simulink model "path_follower_req01"  (R2024a)
settings: Solver=VariableStepAuto  StartTime=0.0  StopTime=10.0  RelTol=1e-3
libraries: simulink x1
settings Model: Creator=rodri  LastModifiedBy=rodri

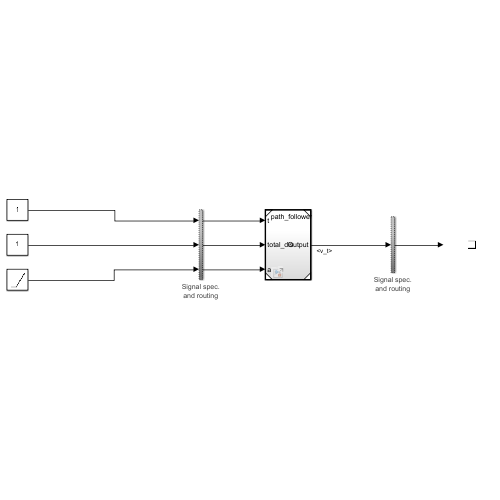
[thumbnail: Simulink's stored preview of the top-level diagram]
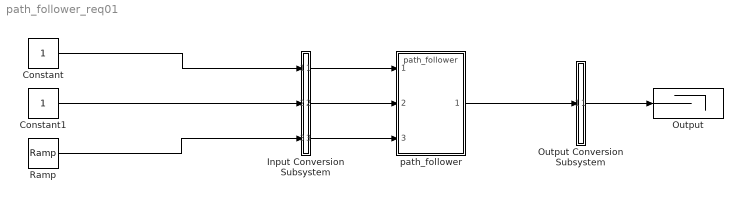
== system path_follower_req01 ==
  Constant : Constant
  Constant1 : Constant
  Input Conversion Subsystem : Subsystem  Tag=__SLT_ICS__  Description=|
      | Signal spec.
      | and routing
      settings: AttributesFormatString=%<Description>
  Output : Terminator
  Output Conversion Subsystem : Subsystem  Tag=__SLT_OCS__  Description=|
      | Signal spec.
      | and routing
      settings: AttributesFormatString=%<Description>
  Ramp : simulink/Sources/Ramp  slope=1  start=0  InitialOutput=0
  path_follower : ModelReference  ModelNameDialog=path_follower  SimulationMode=Normal  ModelReferenceVersion=1.2
  wires:
  Output Conversion Subsystem/1(Outport_1) -> Output/1
  Input Conversion Subsystem/1(Outport_1) -> path_follower/1
  Input Conversion Subsystem/2(Outport_2) -> path_follower/2
  Input Conversion Subsystem/3(Outport_3) -> path_follower/3
  path_follower/1 -> Output Conversion Subsystem/1(Inport_1)
  Constant/1 -> Input Conversion Subsystem/1(Inport_1)
  Constant1/1 -> Input Conversion Subsystem/2(Inport_2)
  Ramp/1 -> Input Conversion Subsystem/3(Inport_3)

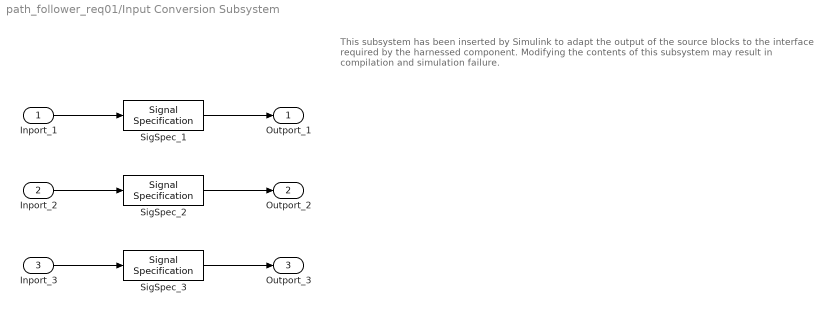
== system path_follower_req01/Input Conversion Subsystem ==
  note: This subsystem has been inserted by Simulink to adapt the output of the source blocks to the interface required by the harnessed component.
      |  Modifying the contents of this subsystem may result in compilation and simulation failure.
  Inport_1 : Inport
  Inport_2 : Inport  Port=2
  Inport_3 : Inport  Port=3
  SigSpec_1 : SignalSpecification  OutDataTypeStr=double  Dimensions=[1]  SampleTime=[0, 0]
  SigSpec_2 : SignalSpecification  OutDataTypeStr=double  Dimensions=[1]  SampleTime=[0, 0]
  SigSpec_3 : SignalSpecification  OutDataTypeStr=double  Dimensions=[1]  SampleTime=[0, 0]
  Outport_1 : Outport
  Outport_2 : Outport  Port=2
  Outport_3 : Outport  Port=3
  wires:
  SigSpec_1/1 -> Outport_1/1
  Inport_1/1 -> SigSpec_1/1
  SigSpec_2/1 -> Outport_2/1
  Inport_2/1 -> SigSpec_2/1
  SigSpec_3/1 -> Outport_3/1
  Inport_3/1 -> SigSpec_3/1

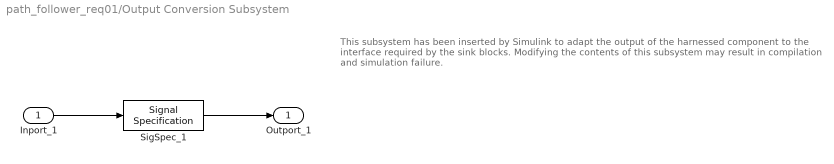
== system path_follower_req01/Output Conversion Subsystem ==
  note: This subsystem has been inserted by Simulink to adapt the output of the harnessed component to the interface required by the sink blocks.
      |  Modifying the contents of this subsystem may result in compilation and simulation failure.
  Inport_1 : Inport
  SigSpec_1 : SignalSpecification  OutDataTypeStr=double  Dimensions=[1]
  Outport_1 : Outport
  wires:
  Inport_1/1 -> SigSpec_1/1
  SigSpec_1/1 -> Outport_1/1
